simulink model "bldcwithoutpid"  (R2016a)
settings: Solver=VariableStepAuto  StartTime=0.0  StopTime=5  RelTol=1e-3
libraries: simulink x6, powerlib x4
settings Model: Creator=prajay  LastModifiedBy=prajay

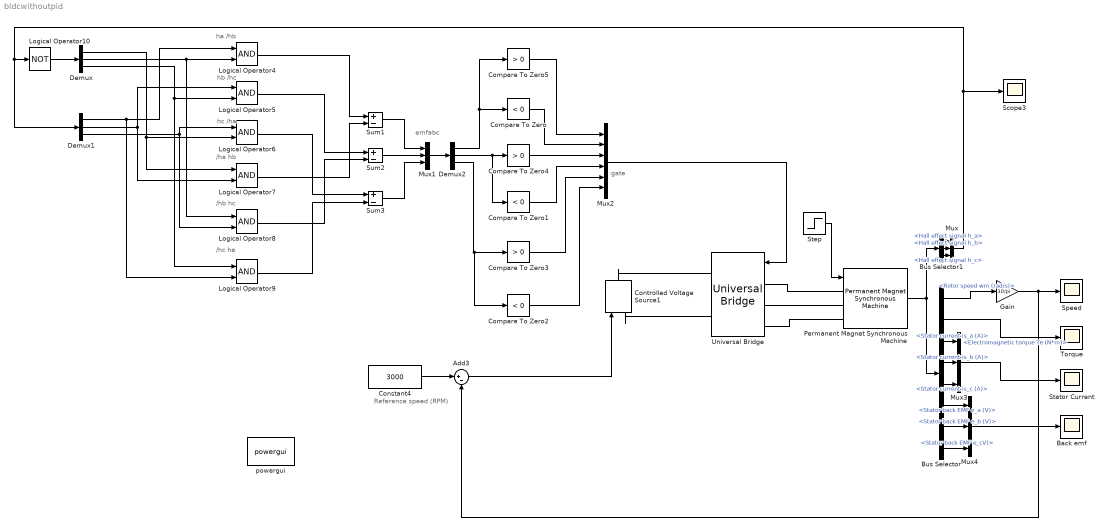
== system bldcwithoutpid ==
  note: gate
  note: emfabc
  note: /hc ha
  note: /hb hc
  note: /ha hb
  note: hc /ha
  note: hb /hc
  note: ha /hb
  note: Reference
      | speed (RPM)
  Add3 : Sum  Inputs=|+-
  Back emf : Scope
  Bus Selector : BusSelector  OutputSignals=Rotor speed wm (rad/s),Electromagnetic torque Te (N*m),Stator current is_a (A),Stator current is_b (A),Stator current is_c (A),Stator back EMF e_a (V),Stator back EMF e_b (V),Stator back EMF e_cV)
  Bus Selector1 : BusSelector  OutputSignals=Hall effect signal h_a,Hall effect signal h_b,Hall effect signal h_c
  Compare To Zero : simulink/Logic and Bit Operations/Compare To Zero  relop=<  OutDataTypeStr=boolean
  Compare To Zero1 : simulink/Logic and Bit Operations/Compare To Zero  relop=<  OutDataTypeStr=boolean
  Compare To Zero2 : simulink/Logic and Bit Operations/Compare To Zero  relop=<  OutDataTypeStr=boolean
  Compare To Zero3 : simulink/Logic and Bit Operations/Compare To Zero  relop=>  OutDataTypeStr=boolean
  Compare To Zero4 : simulink/Logic and Bit Operations/Compare To Zero  relop=>  OutDataTypeStr=boolean
  Compare To Zero5 : simulink/Logic and Bit Operations/Compare To Zero  relop=>  OutDataTypeStr=boolean
  Constant4 : Constant  Value=3000
  Controlled Voltage Source1 : powerlib/Electrical Sources/Controlled Voltage Source  Initialize=on  Source_Type=DC  Amplitude=48  Phase=0  Frequency=0  Measurements=None
  Demux : Demux  Outputs=3
  Demux1 : Demux  Outputs=3
  Demux2 : Demux  Outputs=3
  Gain : Gain  Gain=30/pi
  Logical Operator10 : Logic  Operator=NOT  AllPortsSameDT=off  OutDataTypeStr=boolean
  Logical Operator{4..9} (6 alike) : Logic  AllPortsSameDT=off  OutDataTypeStr=boolean
  Mux{,1,3..4} (4 alike) : Mux  Inputs=3
  Mux2 : Mux  Inputs=6
  Permanent Magnet Synchronous Machine : powerlib/Machines/Permanent Magnet Synchronous Machine  NbPhases=3  FluxDistribution=Trapezoidal  RotorType=Round  MechanicalLoad=Torque Tm  PresetModel=No  ShowDetailedParameters=on  MeasurementBus=off  Resistance=0.25  Inductance=0.32e-3  dqInductances=[8.5e-3,8.5e-3]  La=0.000395  MachineConstant=Voltage Constant (V_peak L-L / krpm)  Flux=0.003581  VoltageCst=6  TorqueCst=0.057296  Flat=120  Mechanical=[0.003 0.0004924 8 0]  PolePairs=4  InitialConditions=[0,0, 0,0]  InitialConditions5ph=[0 0 0 0 0 0]  TsPowergui=0  TsBlock=-1  RefAngle=90 degrees behind phase A axis (modified Park)
  Scope3 : Scope
  Speed : Scope
  Stator Current : Scope
  Step : Step  Time=2.5  After=10  SampleTime=0
  Sum1 : Sum  Inputs=+-  OutDataTypeStr=double
  Sum2 : Sum  Inputs=+-  OutDataTypeStr=double
  Sum3 : Sum  Inputs=+-  OutDataTypeStr=double
  Torque : Scope
  Universal Bridge : powerlib/Power Electronics/Universal Bridge  Arms=3  SnubberResistance=5000  SnubberCapacitance=1e-6  Device=MOSFET / Diodes  Ron=1e-3  Lon=0  ForwardVoltages="[  0  0  ]"  ForwardVoltage=0  GTOparameters=[ 10e-6 , 20e-6 ]  IGBTparameters=[ 1e-6 , 2e-6 ]  Measurements=None  Measurements_2=None  converterType=Rectifier
  powergui : powerlib/powergui  Priority=1  SimulationMode=Continuous  SolverType=Tustin/Backward Euler (TBE)  SampleTime=50e-6  frequency=60  SPID=off  DisableSnubberDevices=off  DisableRonSwitches=off  DisableVfSwitches=off  SwTol=0  DisplayEquations=off  Interpol=off  ExternalGateDelay=off  methode=off  Ts=10  FunctionMessages=off  echomessages=off  HookPort=off  EnableUseOfTLC=off  x0status=blocks  frequencyindice=0  Pbase=100e6  ErrMax=1e-4  Iterations=50  UnitsV=kV  UnitsW=MW  buscounter=0  RestoreLinks=warning  ResistiveCurrentMeasurement=off  Frange=[0:2:500]  Ylog=off  Xlog=on  ShowGrid=off  save=off  variable=ZData  structure=0  ZoomFFT=off  StartTime=0.0  cycles=1  DisplayStyle=1  fundamental=60  FreqAxis=off  MaxFrequency=1000  frequencyindicesteady=1  RmsSteady=1  display=off
  wires:
  Step/1 -> Permanent Magnet Synchronous Machine/1
  Permanent Magnet Synchronous Machine/1 -> Bus Selector1/1, Bus Selector/1
  Bus Selector1/1 -> Mux/1  "<Hall effect signal h_a>"
  Bus Selector1/2 -> Mux/2  "<Hall effect signal h_b>"
  Bus Selector1/3 -> Mux/3  "<Hall effect signal h_c>"
  Mux/1 -> Scope3/1, Demux1/1, Logical Operator10/1
  Logical Operator10/1 -> Demux/1
  Demux1/1 -> Logical Operator9/2, Logical Operator4/1
  Demux/2 -> Logical Operator8/1, Logical Operator4/2
  Demux1/2 -> Logical Operator7/2, Logical Operator5/1
  Demux/3 -> Logical Operator9/1, Logical Operator5/2
  Demux1/3 -> Logical Operator6/1, Logical Operator8/2
  Demux/1 -> Logical Operator7/1, Logical Operator6/2
  Logical Operator4/1 -> Sum1/1
  Logical Operator7/1 -> Sum1/2
  Logical Operator5/1 -> Sum2/1
  Logical Operator8/1 -> Sum2/2
  Logical Operator6/1 -> Sum3/1
  Logical Operator9/1 -> Sum3/2
  Sum1/1 -> Mux1/1
  Sum2/1 -> Mux1/2
  Sum3/1 -> Mux1/3
  Mux1/1 -> Demux2/1
  Demux2/1 -> Compare To Zero/1, Compare To Zero5/1
  Demux2/2 -> Compare To Zero1/1, Compare To Zero4/1
  Demux2/3 -> Compare To Zero2/1, Compare To Zero3/1
  Compare To Zero5/1 -> Mux2/1
  Compare To Zero/1 -> Mux2/2
  Compare To Zero4/1 -> Mux2/3
  Compare To Zero1/1 -> Mux2/4
  Compare To Zero3/1 -> Mux2/5
  Compare To Zero2/1 -> Mux2/6
  Mux2/1 -> Universal Bridge/1
  Bus Selector/2 -> Torque/1  "<Electromagnetic torque Te (N*m)>"
  Bus Selector/1 -> Gain/1  "<Rotor speed wm (rad/s)>"
  Constant4/1 -> Add3/1
  Bus Selector/3 -> Mux3/1  "<Stator current is_a (A)>"
  Bus Selector/4 -> Mux3/2  "<Stator current is_b (A)>"
  Bus Selector/5 -> Mux3/3  "<Stator current is_c (A)>"
  Mux3/1 -> Stator Current/1
  Bus Selector/6 -> Mux4/1  "<Stator back EMF e_a (V)>"
  Bus Selector/8 -> Mux4/3  "<Stator back EMF e_cV)>"
  Bus Selector/7 -> Mux4/2  "<Stator back EMF e_b (V)>"
  Mux4/1 -> Back emf/1
  Add3/1 -> Controlled Voltage Source1/1
  Gain/1 -> Speed/1, Add3/2
  connections:
  Controlled Voltage Source1/RConn1 -- Universal Bridge/RConn1
  Controlled Voltage Source1/LConn1 -- Universal Bridge/RConn2
  Universal Bridge/LConn1 -- Permanent Magnet Synchronous Machine/LConn1
  Universal Bridge/LConn2 -- Permanent Magnet Synchronous Machine/LConn2
  Universal Bridge/LConn3 -- Permanent Magnet Synchronous Machine/LConn3
